simulink model "Lab7_1_sol"  (R2024a)
settings: Solver=ode45  StartTime=0.0  StopTime=8192/100e6  RelTol=1e-3  EnableMultiTasking=on
undefined symbols (not defined in the file): xc7vx485tffg1157, xlfda_numerator
libraries: hdlBasic x4, dspsrcs4 x3, hdlUtilities x1, hdlDSPIP x1, vmcUtilities x1
settings Model: Creator=danielm  LastModifiedBy=sdegala
settings SolverCC: AlgebraicLoopSolver=TrustRegion
settings DataIOCC: LimitDataPoints=on  SaveFormat=Array  ReturnWorkspaceOutputs=off
settings OptimizationCC: LifeSpan=inf
settings DebuggingCC: UnderspecifiedInitializationDetection=Classic  MergeDetectMultiDrivingBlocksExec=none  SolverPrmCheckMsg=warning  UnconnectedInputMsg=warning  UnconnectedOutputMsg=warning  UnconnectedLineMsg=warning  SFUnexpectedBacktrackingDiag=warning  SFNoUnconditionalDefaultTransitionDiag=warning  SFExecutionAtInitializationDiag=none  ArithmeticOperatorsInVariantConditions=warning
settings HardwareCC: ProdBitPerPointer=32  ProdBitPerSizeT=32  ProdBitPerPtrDiffT=32  ProdLargestAtomicFloat=None  ProdIntDivRoundTo=Undefined  ProdEndianess=Unspecified  ProdWordSize=32  ProdHWDeviceType=32-bit Generic
settings ModelReferenceCC: EnableRefExpFcnMdlSchedulingChecks=on  PropagateSignalLabelsOutOfModel=off
settings SFSimCC: SimUseLocalCustomCode=off  CustomCodeUndefinedFunction=UseInterfaceOnly
settings RTWCC: RTWUseLocalCustomCode=off  GPUComputeCapability=3.5
settings CodeAppCC: StateflowObjectComments=on
settings GRTTargetCC: TargetLangStandard=C89/C90 (ANSI)
settings ConfigComp: CovMetricSettings=dw  CovSaveCumulativeToWorkspaceVar=on  CovSaveSingleToWorkspaceVar=on  CovExternalEMLEnable=off  CovSFcnEnable=off

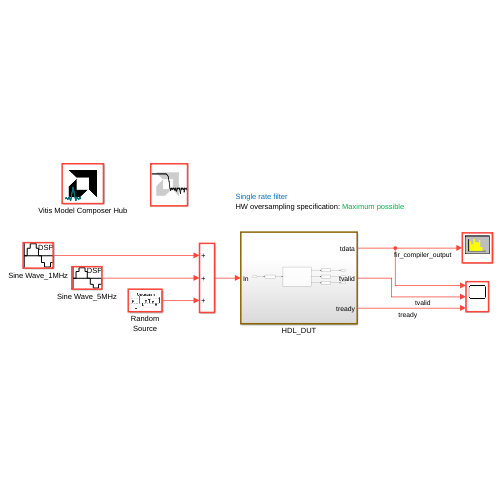
[thumbnail: Simulink's stored preview of the top-level diagram]
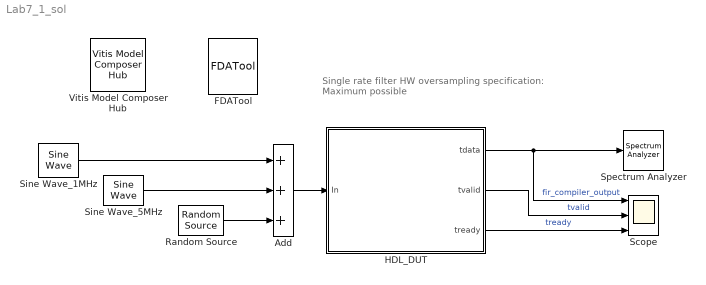
== system Lab7_1_sol ==
  note: Single rate filter
      | HW oversampling specification: Maximum possible
  Add : Sum  Inputs=+++
  FDATool : hdlUtilities/FDATool  block_type=fdatool
      settings: infoedit=FDATool
  HDL_DUT : Subsystem
  Random Source : dspsrcs4/Random Source  SrcType=Gaussian  MinVal=0  MaxVal=1  MeanVal=0  VarVal=1e-5  RepMode=Not repeatable  rawSeed=1  IsInherit=off  SampTime=1/100e6  SampFrame=1  OutComplex=Real  DataType=single  SimulateUsing=Interpreted execution
  Scope : Scope  NumInputPorts=3
  Sine Wave_1MHz : dspsrcs4/Sine Wave  Amplitude=1  Frequency=1e6  Phase=0  SampleMode=Discrete  OutComplex=Real  CompMethod=Trigonometric fcn  TableSize=Speed  SampleTime=1/100e6  SamplesPerFrame=1  ResetState=Restart at time zero  OutputFrames=off  dataType=single  wordLen=16  udDataType=sfix(16)  fracBitsMode=Best precision  numFracBits=15  OutDataTypeStr=single  LastOutDataTypeStr=single
  Sine Wave_5MHz : dspsrcs4/Sine Wave  Amplitude=1  Frequency=5e6  Phase=0  SampleMode=Discrete  OutComplex=Real  CompMethod=Trigonometric fcn  TableSize=Speed  SampleTime=1/100e6  SamplesPerFrame=1  ResetState=Restart at time zero  OutputFrames=off  dataType=single  wordLen=16  udDataType=sfix(16)  fracBitsMode=Best precision  numFracBits=15  OutDataTypeStr=single  LastOutDataTypeStr=single
  Spectrum Analyzer : SpectrumAnalyzer  WindowPosition=[1.000000,1.000000,1280.000000,744.000000,]  Visible=on  ScopeFrameLocation=window  Span=99999.99999999999  StartFrequency=-49999.99999999999  StopFrequency=49999.99999999999  YLimits=[-50.25120223635162,32.58269083372339]  ShowLegend=on
  Vitis Model Composer Hub : vmcUtilities/Vitis Model Composer Hub  Tag=genX  CodeGeneration=off  SubsystemName=HDL_DUT  StartColumn=1  NumberOfColumns=1  TargetDirectory=./code  exportDesign=off  analyzeDesign=off  validateDesignOnHw=off  ExportType=AI Engines  IpVendor=xilinx.com  IpLibrary=hls  IpVersion=1.0  IpHWLanguage=Verilog  AieCompilerOptions={}  AieSimulatorOptions={}  CreateTestbench=off  TestbenchStackSize=10  RunRtlSim=off  RunCSim=off  RunAieSim=off  AieSimTimeout=50000  RunAieSimProfiling=off  LaunchVitisAnalyzer=off  PlotOutput=off  RunX86Sim=off  X86SimTimeout=10  GenHwImage=off  GenLibadfXo=on  GenHwValidationCode=off  PlatformType=Not Specified  HwSystemType=Baremetal  HwValidationTarget=hw  ProjDevice=xc7vx485tffg1157-3  ProjDevicePart=xc7vx485tffg1157-3  SamplePeriod=-1  ClockFrequency=200  DataPathParallelism=1  xilinxfamily=virtex7  part=xc7vx485t  speed=-3  package=ffg1157  directory=./netlist/ip/HDL_DUT/src  testbench=off  incr_netlist=off  synthesis_tool=Vivado  clock_wrapper=Clock Enables  dbl_ovrd=According to Block Masks  dcm_input_clock_period=10  sysclk_period=10  simulink_period=1/100e6  eval_field=0  LogFileName=''  NThreads=4
  wires:
  Sine Wave_5MHz/1 -> Add/2
  Add/1 -> HDL_DUT/1(In)
  HDL_DUT/1(tdata) -> Spectrum Analyzer/1, Scope/1  "fir_compiler_output"
  Random Source/1 -> Add/3
  HDL_DUT/2(tvalid) -> Scope/2  "tvalid"
  HDL_DUT/3(tready) -> Scope/3  "tready"
  Sine Wave_1MHz/1 -> Add/1

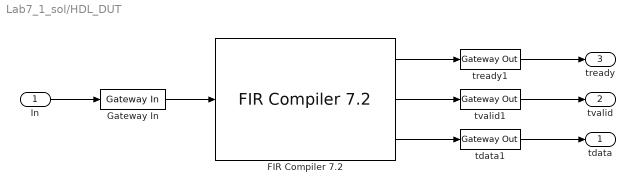
== system Lab7_1_sol/HDL_DUT ==
  In : Inport
  FIR Compiler 7.2 : hdlDSPIP/FIR Compiler 7.2   coefficientvector=double(xlfda_numerator(strcat(bdroot,'/FDATool')))  coefficient_sets=1  coefficient_reload=off  filter_type=Single_Rate  rate_change_type=Fixed_Fractional  interpolation_rate=1  decimation_rate=1  zero_pack_factor=1  channel_sequence=Basic  number_channels=1  pattern_list='P4-0,P4-1,P4-2,P4-3,P4-4'  number_paths=1  ratespecification=Maximum_Possible  sampleperiod=1  hardwareoversamplingrate=5  coefficient_sign=Signed  quantization=Quantize_Only  coefficient_width=16  bestprecision=off  coefficient_fractional_bits=14  coefficient_structure=Inferred  output_rounding_mode=Full_Precision  output_width=16  filter_architecture=Systolic_Multiply_Accumulate  optimization_goal=Area  optimization_list='None'  data_buffer_type=Automatic  coefficient_buffer_type=Automatic  input_buffer_type=Automatic  output_buffer_type=Automatic  preference_for_other_storage=Automatic  multi_column_support=Automatic  columnconfig='99'  inter_column_pipe_length=4  data_has_tlast=Not_Required  m_data_has_tready=off  s_data_has_fifo=off  s_data_has_tuser=Not_Required  m_data_has_tuser=Not_Required  s_config_sync_mode=On_Vector  s_config_method=Single  num_reload_slots=1  has_aclken=off  has_aresetn=off  reset_data_vector=on  trim_axipin_name=on  simulation_type=hybrid_sim  simulation_model=sysgen:xfirv7_2_cmodel  data_path_portlist={ 's_axis_data_tdata', 'm_axis_data_tdata' }  passband_min=0.0  passband_max=0.5  stopband_min=0.5  stopband_max=1.0  filter_selection=1  gui_behaviour='Sysgen_GUI'  data_sign=Signed  data_width=16  data_fractional_bits=0  data_tuser_width=1  wrapper_available=true  ip_wrap_arbitrary_binary_point=true  ip_name=FIR Compiler  ip_version=7.2  dsptool_ready=true  ipcore_usecache=true  ipcore_useipmodelcache=true  port_translation_map={ 'aclken' => 'en', 'aresetn' => 'rst' }  run_core_at_system_period=true  ipcore_xco_need_fpga_part=true  ipcore_fpga_part=[]  XmcBlockStatus=1  maskContainerNames=tabcontainer1  block_type=fir_compiler_v7_2  block_config=sysgen:rodinimport_config  block_width=820  block_height=600
  Gateway In : hdlBasic/Gateway In  gui_display_data_type=Fixed-point  arith_type=Signed (2's comp)  n_bits=16  bin_pt=14  preci_type=Single  exp_width=8  frac_width=24  rows=1  columns=1  quantization="Round  (unbiased: +/- Inf)"  overflow=Saturate  period=1/100e6  UseAsADC=off  ADCChannel='1'  interface=None  automatic_assignment=on  address_offset=hex2dec('00')  intf_name=''  intf_description=''  default_value=0  timing_constraint=None  locs_specified=off  LOCs={}  io_standard={}  inherit_from_input=off  hdl_port=on  XmcBlockStatus=1  maskContainerNames=group4  block_type=gatewayin  block_config=sysgen:gateway_in_config  block_width_w=590  block_height_w=620  block_width=640  block_height=850
  tdata1 : hdlBasic/Gateway Out  inherit_from_input=off  hdl_port=on  rows=1  columns=1  UseAsDAC=off  DACChannel='1'  interface=None  automatic_assignment=on  address_offset=hex2dec('00')  intf_name=''  intf_description=''  timing_constraint=None  locs_specified=off  LOCs={}  io_standard={}  XmcBlockStatus=1  maskContainerNames=group4  block_type=gatewayout  block_config=sysgen:gateway_out_config  block_width_w=590  block_height_w=620  block_width=620  block_height=750
  tready1 : hdlBasic/Gateway Out  inherit_from_input=off  hdl_port=on  rows=1  columns=1  UseAsDAC=off  DACChannel='1'  interface=None  automatic_assignment=on  address_offset=hex2dec('00')  intf_name=''  intf_description=''  timing_constraint=None  locs_specified=off  LOCs={}  io_standard={}  XmcBlockStatus=1  maskContainerNames=group4  block_type=gatewayout  block_config=sysgen:gateway_out_config  block_width_w=590  block_height_w=620  block_width=620  block_height=750
  tvalid1 : hdlBasic/Gateway Out  inherit_from_input=off  hdl_port=on  rows=1  columns=1  UseAsDAC=off  DACChannel='1'  interface=None  automatic_assignment=on  address_offset=hex2dec('00')  intf_name=''  intf_description=''  timing_constraint=None  locs_specified=off  LOCs={}  io_standard={}  XmcBlockStatus=1  maskContainerNames=group4  block_type=gatewayout  block_config=sysgen:gateway_out_config  block_width_w=590  block_height_w=620  block_width=620  block_height=750
  tdata : Outport
  tvalid : Outport  Port=2
  tready : Outport  Port=3
  wires:
  FIR Compiler 7.2/3 -> tdata1/1
  FIR Compiler 7.2/1 -> tready1/1
  In/1 -> Gateway In/1
  FIR Compiler 7.2/2 -> tvalid1/1
  Gateway In/1 -> FIR Compiler 7.2/1
  tdata1/1 -> tdata/1
  tready1/1 -> tready/1
  tvalid1/1 -> tvalid/1
